simulink model "speaker_both"  (R2023a)
settings: Solver=ode45  StartTime=0.0  StopTime=1  MaxStep=1e-5  RelTol=1e-3  EnableMultiTasking=on
InitFcn:
  | %  Table 10.1 pp 167
  | % MKS units
  | 
  | Re=3.36;              % ohms
  | Le = 0.274e-3;     % henries
  | Bl   = 4.9;              % N/A  Newtons/Amp
  | mm = 14.7e-3;      % kg
  | cm  = 0.56e-3;      % m/N
  | rm  = 0.784;          % kg/s
libraries: fl_lib x11, nesl_utility x5, simulink x1
settings Model: Creator=dbenson  LastModifiedBy=ftiong
settings SolverCC: AlgebraicLoopSolver=TrustRegion
settings DataIOCC: LimitDataPoints=on  SaveFormat=Array  SignalLoggingSaveFormat=ModelDataLogs  ReturnWorkspaceOutputs=off
settings OptimizationCC: ExpressionDepthLimit=2147483647  LifeSpan=inf
settings DebuggingCC: UnderspecifiedInitializationDetection=Classic  MergeDetectMultiDrivingBlocksExec=none  SolverPrmCheckMsg=warning  FcnCallInpInsideContextMsg=warning  UnconnectedInputMsg=warning  UnconnectedOutputMsg=warning  UnconnectedLineMsg=warning  StateNameClashWarn=warning  SFUnexpectedBacktrackingDiag=warning  SFNoUnconditionalDefaultTransitionDiag=warning  SFExecutionAtInitializationDiag=none  ArithmeticOperatorsInVariantConditions=warning
settings HardwareCC: ProdBitPerPointer=32  ProdBitPerSizeT=32  ProdBitPerPtrDiffT=32  ProdLargestAtomicFloat=None  ProdIntDivRoundTo=Undefined  ProdEndianess=Unspecified  ProdWordSize=32  ProdHWDeviceType=32-bit Generic
settings ModelReferenceCC: EnableRefExpFcnMdlSchedulingChecks=on  PropagateSignalLabelsOutOfModel=off
settings SFSimCC: SimUseLocalCustomCode=off  CustomCodeUndefinedFunction=UseInterfaceOnly
settings RTWCC: RTWUseLocalCustomCode=off
settings CodeAppCC: StateflowObjectComments=on
settings GRTTargetCC: TargetLangStandard=C89/C90 (ANSI)  CombineOutputUpdateFcns=off  GRTInterface=on
settings ConfigComp: CovMetricSettings=dw  CovSaveCumulativeToWorkspaceVar=on  CovSaveSingleToWorkspaceVar=on  CovExternalEMLEnable=off  CovSFcnEnable=off
settings SimscapeCC: SimscapeNormalizeSystem=off

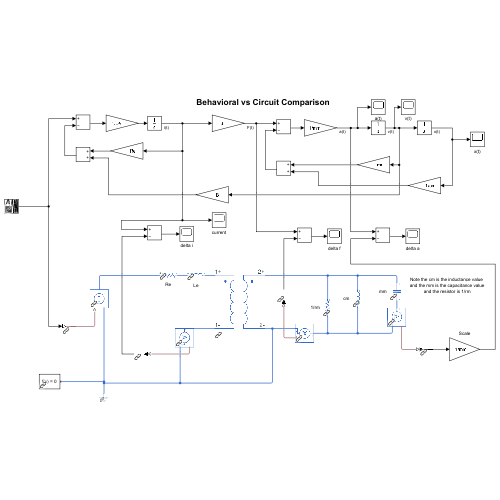
[thumbnail: Simulink's stored preview of the top-level diagram]
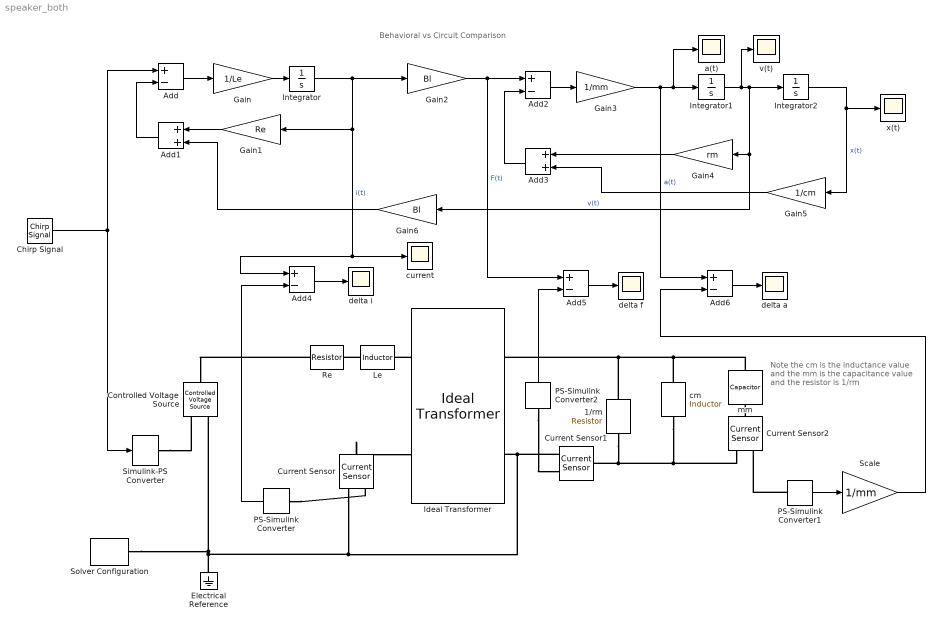
== system speaker_both ==
  note: Behavioral vs Circuit Comparison
  note: Note the cm is the inductance value
      | and the mm is the capacitance value
      | and the resistor is 1/rm
  1/rm : fl_lib/Electrical/Electrical Elements/Resistor  R=1/rm Ohm  i_specify=off  i_priority=High  i=0 A  i_nominal_specify=off  i_nominal_unit=A  i_nominal_value=1  v_specify=off  v_priority=High  v=0 V  v_nominal_specify=off  v_nominal_unit=V  v_nominal_value=1
  Add{,2,4..6} (5 alike) : Sum  Inputs=+-
  Add1 : Sum
  Add3 : Sum
  Chirp Signal : simulink/Sources/Chirp Signal  f1=10  T=1  f2=1000
  Controlled Voltage Source : fl_lib/Electrical/Electrical Sources/Controlled Voltage Source
  Current Sensor : fl_lib/Electrical/Electrical Sensors/Current Sensor
  Current Sensor1 : fl_lib/Electrical/Electrical Sensors/Current Sensor
  Current Sensor2 : fl_lib/Electrical/Electrical Sensors/Current Sensor
  Electrical Reference : fl_lib/Electrical/Electrical Elements/Electrical Reference
  Gain : Gain  Gain=1/Le
  Gain1 : Gain  Gain=Re
  Gain2 : Gain  Gain=Bl
  Gain3 : Gain  Gain=1/mm
  Gain4 : Gain  Gain=rm
  Gain5 : Gain  Gain=1/cm
  Gain6 : Gain  Gain=Bl
  Ideal Transformer : fl_lib/Electrical/Electrical Elements/Ideal Transformer  n=Bl  i1_specify=off  i1_priority=High  i1=0 A  i1_nominal_specify=off  i1_nominal_unit=A  i1_nominal_value=1  v1_specify=off  v1_priority=High  v1=0 V  v1_nominal_specify=off  v1_nominal_unit=V  v1_nominal_value=1  i2_specify=off  i2_priority=High  i2=0 A  i2_nominal_specify=off  i2_nominal_unit=A  i2_nominal_value=1  v2_specify=off  v2_priority=High  v2=0 V  v2_nominal_specify=off  v2_nominal_unit=V  v2_nominal_value=1
  Integrator : Integrator
  Integrator1 : Integrator
  Integrator2 : Integrator
  Le : fl_lib/Electrical/Electrical Elements/Inductor  l=Le H  r=0 Ohm  g=0 1/Ohm  i_specify=off  i_priority=High  i=0 A  i_nominal_specify=off  i_nominal_unit=A  i_nominal_value=1  v_specify=off  v_priority=High  v=0 V  v_nominal_specify=off  v_nominal_unit=V  v_nominal_value=1  i_L_specify=off  i_L_priority=High  i_L=0 A  i_L_nominal_specify=off  i_L_nominal_unit=A  i_L_nominal_value=1
  PS-Simulink Converter : nesl_utility/PS-Simulink Converter  PhysicalDomain=network_engine_domain  SubClassName=ps_output  LeftPortType=input  RightPortType=output  PseudoPeriodic=off  Frequencies=[]  VectorFormat=1-D array  Unit=1  AffineConversion=off
  PS-Simulink Converter1 : nesl_utility/PS-Simulink Converter  PhysicalDomain=network_engine_domain  SubClassName=ps_output  LeftPortType=input  RightPortType=output  PseudoPeriodic=off  Frequencies=[]  VectorFormat=1-D array  Unit=1  AffineConversion=off
  PS-Simulink Converter2 : nesl_utility/PS-Simulink Converter  PhysicalDomain=network_engine_domain  SubClassName=ps_output  LeftPortType=input  RightPortType=output  PseudoPeriodic=off  Frequencies=[]  VectorFormat=1-D array  Unit=1  AffineConversion=off
  Re : fl_lib/Electrical/Electrical Elements/Resistor  R=Re Ohm  i_specify=off  i_priority=High  i=0 A  i_nominal_specify=off  i_nominal_unit=A  i_nominal_value=1  v_specify=off  v_priority=High  v=0 V  v_nominal_specify=off  v_nominal_unit=V  v_nominal_value=1
  Scale : Gain  Gain=1/mm
  Simulink-PS Converter : nesl_utility/Simulink-PS Converter  PhysicalDomain=network_engine_domain  SubClassName=ps_input  LeftPortType=input  RightPortType=output  PseudoPeriodic=off  Frequencies=[]  NoiseDistribution=none  NoiseParameters=[]  Unit=1  AffineConversion=off  FilteringAndDerivatives=zero  SimscapeFilterOrder=1  InputFilterTimeConstant=0.001  UdotUserProvided=1
  Solver Configuration : nesl_utility/Solver Configuration  PhysicalDomain=network_engine_domain  SubClassName=solver  LeftPortType=input  RightPortType=generic  Tones=[]  Harmonics=[]  SimulateNoise=off  Profile=off  UseLocalSampling=off  EnableSwitchedLinearOptims=on  FrequencyDomain=off  UseCCode=off  RelTol=0.001  AbsTol=1e-06  MinStep=1e-09  ToWorkspace=off  RevertToSquareIcSolve=off  NumHomotopyIterations=100  PhasorMode=off  PhasorModeNumHarmonics=1  ConsistencySolver=NEWTON_FTOL  IndexReductionMethod=DerivativeReplacement  DoDC=off  ResidualTolerance=1e-09  ConsistencyTolSource=GLOBAL  ConsistencyAbsTol=0.001  ConsistencyRelTol=0.001  ConsistencyTolFactor=0.001  UseLocalSolver=off  LocalSolverChoice=NE_BACKWARD_EULER_ADVANCER  ResolveIndetEquations=on  FunctionEvalNumThread=1  LocalSolverSampleTime=0.001  DoFixedCost=off  MaxNonlinIter=3  MaxModeIter=2  ComputeImpulses=off  ImpulseIterations=2  LinearAlgebra=Sparse  LinearAlgebraNumThread=0  EquationFormulation=NE_TIME_EF  DelaysMemoryBudget=1024  AutomaticFiltering=on  FilteringTimeConstant=0.001  PartitionStorageMethod=AS_NEEDED  PartitionMemoryBudget=1024  PartitionMethod=FAST
  a(t) : Scope
  cm : fl_lib/Electrical/Electrical Elements/Inductor  l=cm H  r=0 Ohm  g=0 1/Ohm  i_specify=off  i_priority=High  i=0 A  i_nominal_specify=off  i_nominal_unit=A  i_nominal_value=1  v_specify=off  v_priority=High  v=0 V  v_nominal_specify=off  v_nominal_unit=V  v_nominal_value=1  i_L_specify=off  i_L_priority=High  i_L=0 A  i_L_nominal_specify=off  i_L_nominal_unit=A  i_L_nominal_value=1
  current : Scope
  delta a : Scope
  delta f : Scope
  delta i : Scope
  mm : fl_lib/Electrical/Electrical Elements/Capacitor  c=mm F  r=0 Ohm  g=0 1/Ohm  i_specify=off  i_priority=High  i=0 A  i_nominal_specify=off  i_nominal_unit=A  i_nominal_value=1  v_specify=off  v_priority=High  v=0 V  v_nominal_specify=off  v_nominal_unit=V  v_nominal_value=1  vc_specify=off  vc_priority=High  vc=0 V  vc_nominal_specify=off  vc_nominal_unit=V  vc_nominal_value=1
  v(t) : Scope
  x(t) : Scope
  wires:
  Add/1 -> Gain/1
  Gain/1 -> Integrator/1
  Integrator/1 -> Gain2/1, Gain1/1, current/1, Add4/1  "i(t)"
  Add1/1 -> Add/2
  Gain1/1 -> Add1/1
  Gain2/1 -> Add2/1, Add5/1  "F(t)"
  Add2/1 -> Gain3/1
  Gain3/1 -> Add6/1, Integrator1/1, a(t)/1  "a(t)"
  Integrator1/1 -> v(t)/1, Integrator2/1, Gain4/1, Gain6/1  "v(t)"
  Integrator2/1 -> x(t)/1, Gain5/1  "x(t)"
  Add3/1 -> Add2/2
  Gain4/1 -> Add3/1
  Gain5/1 -> Add3/2
  Gain6/1 -> Add1/2
  Chirp Signal/1 -> Simulink-PS Converter/1, Add/1
  Add4/1 -> delta i/1
  Add5/1 -> delta f/1
  Scale/1 -> Add6/2
  Add6/1 -> delta a/1
  PS-Simulink Converter1/1 -> Scale/1
  PS-Simulink Converter2/1 -> Add5/2
  PS-Simulink Converter/1 -> Add4/2
  connections:
  Simulink-PS Converter/RConn1 -- Controlled Voltage Source/RConn1
  Re/LConn1 -- Controlled Voltage Source/LConn1
  Le/LConn1 -- Re/RConn1
  Ideal Transformer/LConn1 -- Le/RConn1
  Current Sensor/LConn1 -- Ideal Transformer/LConn2
  PS-Simulink Converter/LConn1 -- Current Sensor/RConn1
  1/rm/LConn1 -- mm/LConn1 -- cm/LConn1 -- Ideal Transformer/RConn1
  Electrical Reference/LConn1 -- Ideal Transformer/RConn2 -- Current Sensor1/RConn2 -- Current Sensor/RConn2 -- Controlled Voltage Source/RConn2 -- Solver Configuration/RConn1
  cm/RConn1 -- 1/rm/RConn1 -- Current Sensor1/LConn1 -- Current Sensor2/RConn2
  Current Sensor2/LConn1 -- mm/RConn1
  PS-Simulink Converter1/LConn1 -- Current Sensor2/RConn1
  PS-Simulink Converter2/LConn1 -- Current Sensor1/RConn1
